simulink model "lab7_reglare_turatie_slx"  (R2023b)
settings: Solver=ode45  StartTime=0.0  StopTime=15  MaxStep=1e-3  RelTol=1e-5
undefined symbols (not defined in the file or in its folder): sigbuilder_block
settings Model: Creator=Daniela  LastModifiedBy=Daniela

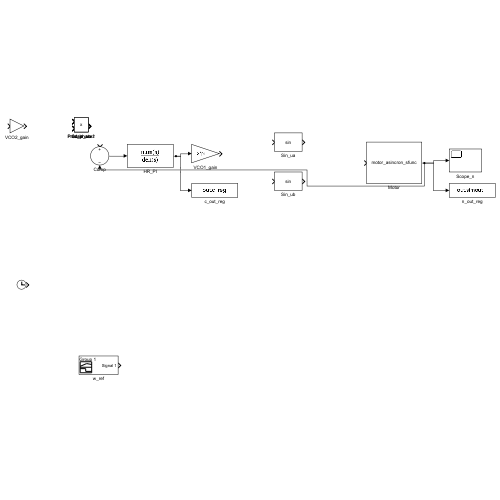
[thumbnail: Simulink's stored preview of the top-level diagram]
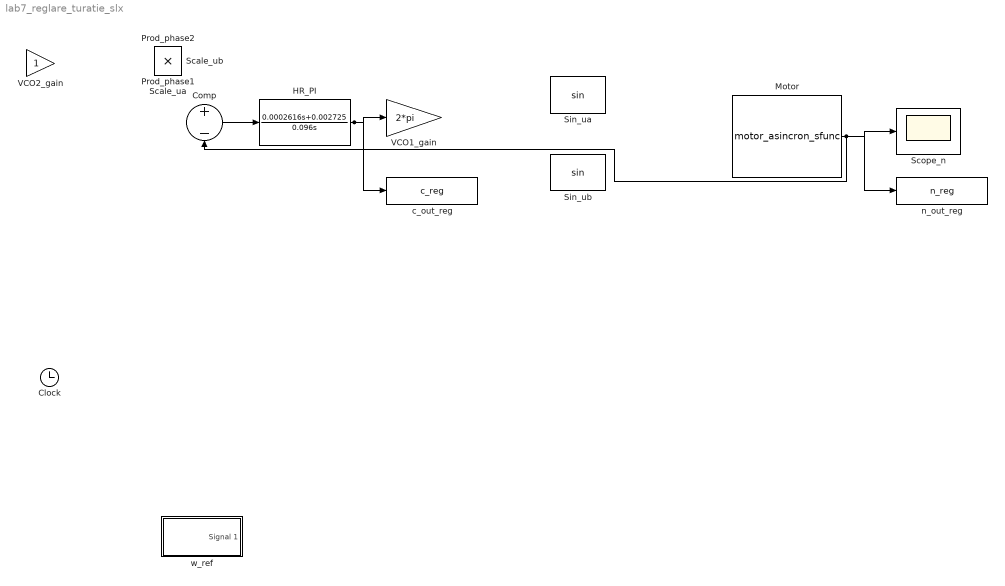
== system lab7_reglare_turatie_slx ==
  Clock : Clock
  Comp : Sum  Inputs=+-
  HR_PI : TransferFcn  Numerator=[0.0002616 0.002725]  Denominator=[0.096 0]
  Motor : M-S-Function  FunctionName=motor_asincron_sfunc
  Prod_phase1 : Product
  Prod_phase2 : Product
  Scale_ua : Product
  Scale_ub : Product
  Scope_n : Scope
  Sin_ua : Trigonometry
  Sin_ub : Trigonometry
  VCO1_gain : Gain  Gain=2*pi
  VCO2_gain : Gain
  c_out_reg : ToWorkspace  VariableName=c_reg  SampleTime=-1
  n_out_reg : ToWorkspace  VariableName=n_reg  SampleTime=-1
  w_ref : Subsystem  Tag=STV Subsys  LoadFcn=sigbuilder_block('load');  StartFcn=sigbuilder_block('start');  StopFcn=sigbuilder_block('stop');  ClipboardFcn=sigbuilder_block('clipboard');  mask(Sigbuilder block){tuvar=[0:10]}
      mask help: Simulink:masks:SigbuilderBlock_MD
      mask init:
      | if ~strcmp(get_param(bdroot(gcbh),'SimulationStatus'),'stopped') tuvar = sigbuilder_block('maskInit'); end
      settings: CopyFcn=sigbuilder_block('copy');  DeleteFcn=sigbuilder_block('delete');  ModelCloseFcn=sigbuilder_block('modelClose');  PreSaveFcn=sigbuilder_block('preSave');  PauseFcn=sigbuilder_block('pause');  ContinueFcn=sigbuilder_block('continue');  NameChangeFcn=sigbuilder_block('namechange');  OpenFcn=sigbuilder_block('open',[437.6 199.2 550.4 400 ]);  CloseFcn=sigbuilder_block('close');
      mask Display: plot(0, 0, 100, 100,[2, 2, 32, 32, 2], [68, 8, 8, 68, 68],[32, 2], [38, 38], [32, 19, 2],[53, 60, 44], [32, 17, 17, 2],[16, 16, 31, 31]);txt = getActiveGroup(gcbh);text(2, 100, txt,'verticalAlignment', 'top');
  wires:
  Comp/1 -> HR_PI/1
  HR_PI/1 -> VCO1_gain/1, c_out_reg/1
  Motor/1 -> Scope_n/1, n_out_reg/1, Comp/2

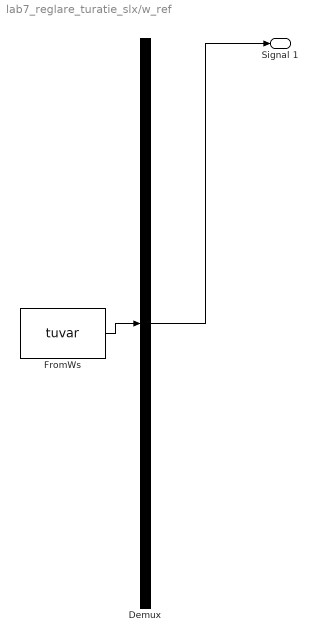
== system lab7_reglare_turatie_slx/w_ref ==
  Demux : Demux  Tag=STV Demux  Outputs=1
      settings: DisplayOption=none
  FromWs : FromWorkspace  Tag=STV FromWs  VariableName=tuvar
      SigBuilderData=|
      | common.afterFinalStr = 'Extrapolate'
      | common.sampleTime = 0
      | dataSet.timeRange = [0 10]
      | dataSet.name = 'Group 1'
      | sbobj.Groups.Name = 'Group 1'
      | sbobj.Groups.Signals.Name = 'Signal 1'
      | sbobj.Groups.Signals.XData = [0 4 4 6 6 10]
      | sbobj.Groups.Signals.YData = [0 0 1 1 0 0]
  Signal 1 : Outport  Tag=STV Outport
  wires:
  FromWs/1 -> Demux/1
  Demux/1 -> Signal 1/1
